simulink model "OFDMTxRx221121"  (R2017b)
settings: Solver=VariableStepAuto  StartTime=0.0  StopTime=10  RelTol=1e-3
InitFcn:
  | Ts = 1e-6;
  | simParams.Ts = Ts;
  | simParams.TsTx = Ts;
  | simParams.TsRx = Ts;
  | simParams.nFFT = 1024;
  | simParams.lengthCP = 128;
  | nFFT = simParams.nFFT;
  | simParams.NSubcarriers = 398;
  | simParams.windowing = 16;
undefined symbols (not defined in the file): fft_size, i
libraries: hdlsllib x34, simulink x26, simulink_need_slupdate x17, dspmathops x5, dspxfrm3 x3, dspsigops x2, commdigbbndam3 x1, commrflib2 x1, commseqgen3 x1
(part 1 of 2)
settings Model: PauseTimes=1  Creator=Pigrit  LastModifiedBy=trainee

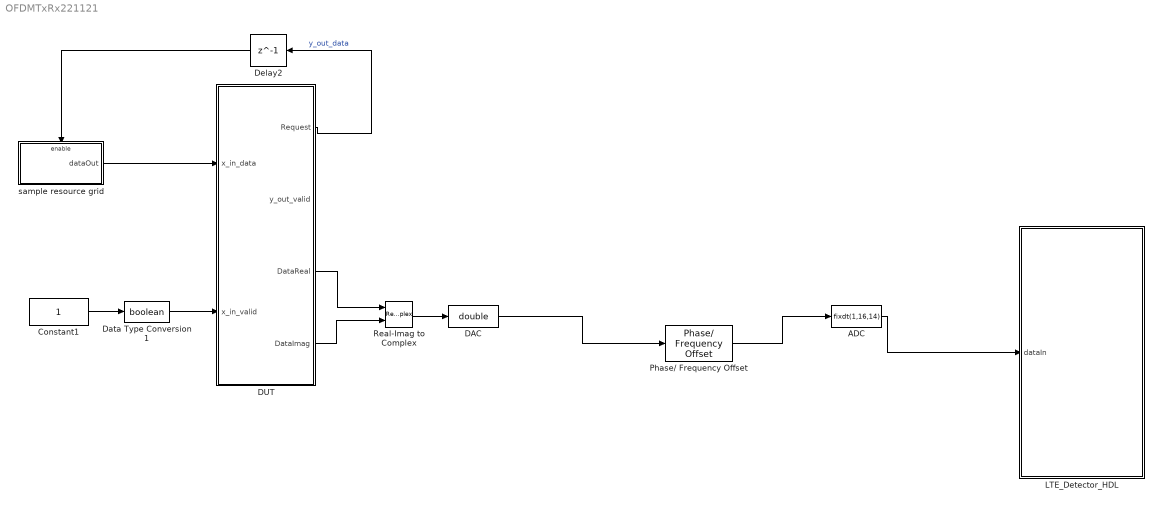
== system OFDMTxRx221121 ==
  ADC : DataTypeConversion  OutDataTypeStr=fixdt(1,16,14)  RndMeth=Nearest
  Constant1 : Constant  OutDataTypeStr=boolean  SampleTime=simParams.Ts
  DAC : DataTypeConversion  OutDataTypeStr=double  RndMeth=Nearest
  DUT : Subsystem  TreatAsAtomicUnit=on
  Data Type Conversion1 : DataTypeConversion  OutDataTypeStr=boolean
  Delay2 : Delay  DelayLength=1  InitialCondition=0  InputProcessing=Columns as channels (frame based)
  LTE_Detector_HDL : Subsystem
  Phase/ Frequency Offset : commrflib2/Phase// Frequency Offset  phaseOffset=0  freqPort=off  freqOffset=0
      settings: SourceProductName=Communications System Toolbox
  Real-Imag to Complex : RealImagToComplex
  sample resource grid : Subsystem
  wires:
  DUT/3(DataReal) -> Real-Imag to Complex/1
  Delay2/1 -> sample resource grid/Enable
  Data Type Conversion1/1 -> DUT/2(x_in_valid)
  Constant1/1 -> Data Type Conversion1/1
  DUT/1(Request) -> Delay2/1  "y_out_data"
  sample resource grid/1(dataOut) -> DUT/1(x_in_data)
  DUT/4(DataImag) -> Real-Imag to Complex/2
  Real-Imag to Complex/1 -> DAC/1
  ADC/1 -> LTE_Detector_HDL/1(dataIn)
  Phase/ Frequency Offset/1 -> ADC/1
  DAC/1 -> Phase/ Frequency Offset/1

== system OFDMTxRx221121/DUT ==
  x_in_data : Inport
  x_in_valid : Inport  Port=2
  "symmetric " : Subsystem
  Request : Outport
  y_out_valid : Outport  Port=2
  DataReal : Outport  Port=3
  DataImag : Outport  Port=4
  wires:
  x_in_valid/1 -> "symmetric "/Enable, y_out_valid/1
  x_in_data/1 -> "symmetric "/1(x_in)
  "symmetric "/1(y_out) -> Request/1
  "symmetric "/2(Data1) -> DataReal/1
  "symmetric "/3(Data2) -> DataImag/1

== system OFDMTxRx221121/LTE_Detector_HDL ==
  dataIn : Inport
  Buffer : Buffer  N=1000  OutputFrames=off
  Constellation Diagram : ConstellationDiagram
  Delay1 : Delay  DelayLength=11  InitialCondition=0
  Delay2 : Delay  DelayLength=1196  InitialCondition=0
  FFT : Subsystem
  Frequency_Correction : Subsystem
  Frequency_Correction1 : Subsystem
  Frequency_Correction2 : Subsystem
  Frequency_Estimation : Subsystem
  Frequency_Estimation1 : Subsystem
  Frequency_Estimation2 : Subsystem
  Number of subcarriers : Constant  Value=0  OutDataTypeStr=fixdt(0,12,0)  SampleTime=Ts
  Scope : Scope  NumInputPorts=3
  Spectrum Analyzer : SpectrumAnalyzer
  Переформирование отсчетов : Subsystem
  Подстройка по фазе : Subsystem
  Стробирование сигнала на nFFT отсчетов : Subsystem
  Эквалайзинг забита только формула : Subsystem
  wires:
  Стробирование сигнала на nFFT отсчетов/1(dataOut) -> FFT/1(dataIn)
  Стробирование сигнала на nFFT отсчетов/2(ValidOut) -> FFT/2(validIn)
  Buffer/1 -> Constellation Diagram/1
  Переформирование отсчетов/3(AngOut) -> Подстройка по фазе/2(AngIn)
  Переформирование отсчетов/4(ValidOut) -> Подстройка по фазе/3("ValidIn "), Эквалайзинг забита только формула/2("ValidIn ")
  Подстройка по фазе/1(Out1) -> Buffer/1
  Переформирование отсчетов/1("PureSig ") -> Подстройка по фазе/1(PureSigIn)
  dataIn/1 -> Spectrum Analyzer/1, Delay2/1, Frequency_Estimation1/1(data)
  FFT/1(dataOut) -> Переформирование отсчетов/1(In1)
  FFT/2(validOut) -> Переформирование отсчетов/2(In2)
  Переформирование отсчетов/2(MagOut) -> Эквалайзинг забита только формула/1(MagIn)
  Frequency_Estimation1/2(MiddlePoint) -> Scope/2, Delay1/1
  Delay2/1 -> Scope/3, Frequency_Correction1/1(dataIn)
  Frequency_Correction1/1(dataOut) -> Стробирование сигнала на nFFT отсчетов/1(In1)
  Delay1/1 -> Стробирование сигнала на nFFT отсчетов/2(In2)
  Frequency_Estimation1/1(freqEst) -> Scope/1, Frequency_Correction1/2(freq)

== system OFDMTxRx221121/sample resource grid ==
  request1 : EnablePort
  PN Sequence Generator : commseqgen3/PN Sequence Generator  poly='z^23+z^21+z^17 + z^11 + z^5 +1'  ini_sta=[0 1 1 0 0 1 0 0 0 0 1 0 1 1 0 0 1 0 0 1 0 0 1]  outBitMaskSource=Dialog parameter  shift=0  outVarSiz=off  maxOutSizeMode=Dialog parameter  maxOutSize=[10 1]  Ts=simParams.Ts  sampPerFrame=1  reset=off  bitPackedOutputs=on  outDataType=boolean  numPackedBits=6  bitPackDataSigned=off  bitPackedOutDType=Smallest integer
      settings: SourceProductName=Communications System Toolbox
  dataOut : Outport
  wires:
  PN Sequence Generator/1 -> dataOut/1

== system OFDMTxRx221121/DUT/symmetric  ==
  x_in : Inport
  Enable : EnablePort
  Add CP and windowing : Subsystem
  Complex to Real-Imag : ComplexToRealImag
  IFFT : Subsystem
  Scope : Scope  NumInputPorts=2
  Scope1 : Scope  NumInputPorts=2
  fORM1 : Subsystem
  y_out1 : Scope  NumInputPorts=2
  "Сдвиг в симметричный вид " : Subsystem
  y_out : Outport  InitialOutput=0
  Data1 : Outport  Port=2  InitialOutput=0
  Data2 : Outport  Port=3  InitialOutput=0
  wires:
  fORM1/1(dataRequest) -> y_out/1
  x_in/1 -> fORM1/1(dataIn)
  Add CP and windowing/1(Out1) -> Complex to Real-Imag/1
  Complex to Real-Imag/1 -> Data2/1
  IFFT/1(dataOut) -> Scope/1, Add CP and windowing/1(In1)
  Complex to Real-Imag/2 -> Data1/1
  "Сдвиг в симметричный вид "/1(dataOut) -> Scope1/1, IFFT/1(dataIn)
  "Сдвиг в симметричный вид "/2(validOut) -> Scope1/2, IFFT/2(validIn)
  IFFT/2(validOut) -> Scope/2, Add CP and windowing/2(In2)
  fORM1/2(dataOut) -> y_out1/1, "Сдвиг в симметричный вид "/1(dataIn)
  fORM1/3(validOut) -> y_out1/2, "Сдвиг в симметричный вид "/2(validIn)

== system OFDMTxRx221121/LTE_Detector_HDL/FFT ==
  note: Set input of FFT to input wordlength + FFT growth to allow
      | the output of the FFT to scale. Maximum bit growth is equal
      | to log2(nFFT).
  dataIn : Inport
  validIn : Inport  Port=2
  Data Type Conversion : DataTypeConversion  OutDataTypeStr=fixdt(1,18,10)  RndMeth=Round
  Delay{1..2,4..5} (4 alike) : Delay  DelayLength=1  InitialCondition=0  InputProcessing=Columns as channels (frame based)
  FFT HDL Optimized : dspxfrm3/FFT HDL Optimized  FFTLength=1024  Architecture=Streaming Radix 2^2  ComplexMultiplication=Use 3 multipliers and 5 adders  BitReversedOutput=off  BitReversedInput=off  Normalize=off  SimulateUsing=Code generation  RoundingMethod=Floor  ResetInputPort=off  StartOutputPort=off  EndOutputPort=off
      settings: SourceProductName=DSP System Toolbox  SourceProductBaseCode=DS
  Signal Specification : SignalSpecification  Dimensions=1
  Signal Specification1 : SignalSpecification  Dimensions=1
  dataOut : Outport
  validOut : Outport  Port=2
  wires:
  Signal Specification1/1 -> FFT HDL Optimized/2
  Signal Specification/1 -> FFT HDL Optimized/1
  FFT HDL Optimized/2 -> Delay5/1
  FFT HDL Optimized/1 -> Delay4/1
  Delay4/1 -> Data Type Conversion/1
  Delay2/1 -> Signal Specification1/1
  dataIn/1 -> Delay1/1
  validIn/1 -> Delay2/1
  Delay1/1 -> Signal Specification/1
  Data Type Conversion/1 -> dataOut/1
  Delay5/1 -> validOut/1

== system OFDMTxRx221121/LTE_Detector_HDL/Frequency_Correction ==
  note: This subsystem corrects the frequency offset using an Numerically Controller Oscillator (NCO) and a conjugate multiplication.
  dataIn : Inport
  freq : Inport  Port=2
  Data Type Conversion : DataTypeConversion  OutDataTypeStr=fixdt(1,16,15)  RndMeth=Nearest
  Delay{1..6} (6 alike) : Delay  DelayLength=1  InitialCondition=0  UseCircularBuffer=on
  Gain : Gain  Gain=2^9  OutDataTypeStr=int16
  NCO HDL Optimized : dspsigops/NCO HDL Optimized  PhaseIncrementSource=Input port  PhaseIncrement=100  PhaseOffsetSource=Property  PhaseOffset=0  DitherSource=Property  NumDitherBits=4  PhaseQuantization=on  NumQuantizerAccumulatorBits=12  LUTCompress=on  ResetAction=off  ValidInputPort=off  Waveform=Complex exponential  PhasePort=off  SimulateUsing=Code generation  AccumulatorWL=16  OutputDataType=Binary point scaling  OutputWL=16  OutputFL=14
      settings: SourceProductName=DSP System Toolbox  SourceProductBaseCode=DS
  Product1 : Product
  Scope : Scope  NumInputPorts=2
  Signal Spec : SignalSpecification  Dimensions=1
  Unit Delay Enabled : simulink_need_slupdate/Unit Delay Enabled  vinit=0.0  tsamp=-1
      settings: SourceProductName=Simulink  SourceProductBaseCode=SL
  complexConjugate : Math  Operator=conj  SaturateOnIntegerOverflow=on
  dataOut : Outport
  wires:
  complexConjugate/1 -> Delay3/1
  NCO HDL Optimized/2 -> Unit Delay Enabled/2
  dataIn/1 -> Delay2/1
  Product1/1 -> Delay4/1
  NCO HDL Optimized/1 -> Unit Delay Enabled/1
  Unit Delay Enabled/1 -> complexConjugate/1
  Data Type Conversion/1 -> Delay1/1
  Delay2/1 -> Scope/2, Product1/1
  Delay1/1 -> dataOut/1
  Delay4/1 -> Data Type Conversion/1
  Delay3/1 -> Scope/1, Product1/2
  Gain/1 -> Delay5/1
  freq/1 -> Delay6/1
  Delay6/1 -> Gain/1
  Signal Spec/1 -> NCO HDL Optimized/1
  Delay5/1 -> Signal Spec/1

== system OFDMTxRx221121/LTE_Detector_HDL/Frequency_Correction1 ==
  note: This subsystem corrects the frequency offset using an Numerically Controller Oscillator (NCO) and a conjugate multiplication.
  dataIn : Inport
  freq : Inport  Port=2
  Data Type Conversion : DataTypeConversion  OutDataTypeStr=fixdt(1,16,15)  RndMeth=Nearest
  Delay{1..6} (6 alike) : Delay  DelayLength=1  InitialCondition=0  UseCircularBuffer=on
  Gain : Gain  Gain=2^9  OutDataTypeStr=int16
  NCO HDL Optimized : dspsigops/NCO HDL Optimized  PhaseIncrementSource=Input port  PhaseIncrement=100  PhaseOffsetSource=Property  PhaseOffset=0  DitherSource=Property  NumDitherBits=4  PhaseQuantization=on  NumQuantizerAccumulatorBits=12  LUTCompress=on  ResetAction=off  ValidInputPort=off  Waveform=Complex exponential  PhasePort=off  SimulateUsing=Code generation  AccumulatorWL=16  OutputDataType=Binary point scaling  OutputWL=16  OutputFL=14
      settings: SourceProductName=DSP System Toolbox  SourceProductBaseCode=DS
  Product1 : Product
  Scope : Scope  NumInputPorts=2
  Signal Spec : SignalSpecification  Dimensions=1
  Unit Delay Enabled : simulink_need_slupdate/Unit Delay Enabled  vinit=0.0  tsamp=-1
      settings: SourceProductName=Simulink  SourceProductBaseCode=SL
  complexConjugate : Math  Operator=conj  SaturateOnIntegerOverflow=on
  dataOut : Outport
  wires:
  complexConjugate/1 -> Delay3/1
  NCO HDL Optimized/2 -> Unit Delay Enabled/2
  dataIn/1 -> Delay2/1
  Product1/1 -> Delay4/1
  NCO HDL Optimized/1 -> Unit Delay Enabled/1
  Unit Delay Enabled/1 -> complexConjugate/1
  Data Type Conversion/1 -> Delay1/1
  Delay2/1 -> Scope/2, Product1/1
  Delay1/1 -> dataOut/1
  Delay4/1 -> Data Type Conversion/1
  Delay3/1 -> Scope/1, Product1/2
  Gain/1 -> Delay5/1
  freq/1 -> Delay6/1
  Delay6/1 -> Gain/1
  Signal Spec/1 -> NCO HDL Optimized/1
  Delay5/1 -> Signal Spec/1

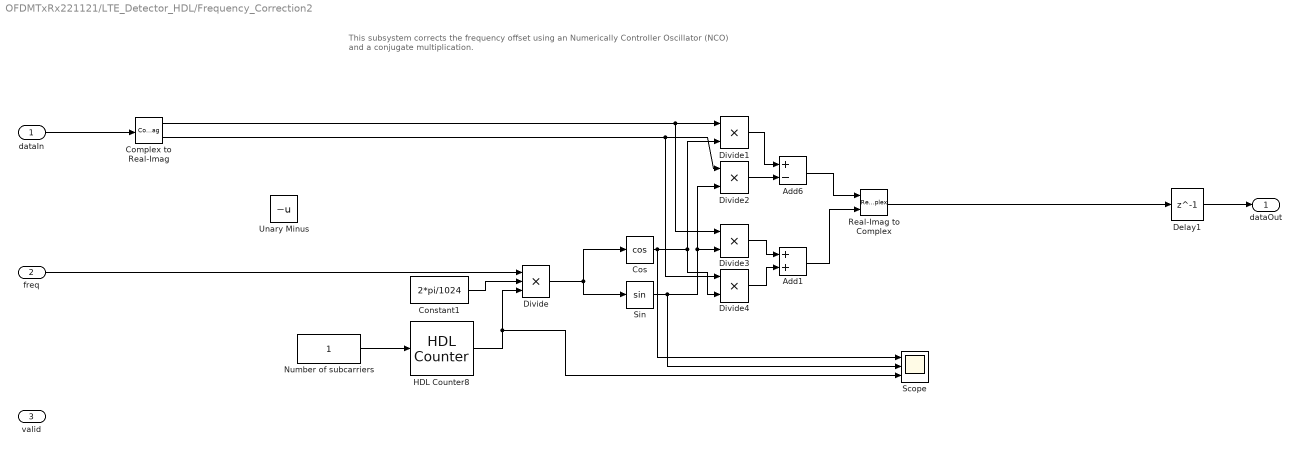
== system OFDMTxRx221121/LTE_Detector_HDL/Frequency_Correction2 ==
  note: This subsystem corrects the frequency offset using an Numerically Controller Oscillator (NCO) and a conjugate multiplication.
  dataIn : Inport
  freq : Inport  Port=2
  "valid " : Inport  Port=3
  Add1 : Sum
  Add6 : Sum  Inputs=+-
  Complex to Real-Imag : ComplexToRealImag
  Constant1 : Constant  Value=2*pi/1024  SampleTime=simParams.Ts
  Cos : Trigonometry  Operator=cos
  Delay1 : Delay  DelayLength=1  InitialCondition=0  UseCircularBuffer=on
  Divide : Product  Inputs=***  SaturateOnIntegerOverflow=on  RndMeth=Zero
  Divide{1..4} (4 alike) : Product  Inputs=**  SaturateOnIntegerOverflow=on  RndMeth=Zero
  HDL Counter8 : hdlsllib/Sources/HDL Counter  CountType=Count limited  CountInit=0  CountStep=1  CountMax=1023  CountFromType=Initial value  CountFrom=0  CountResetPort=off  CountLoadPort=off  CountEnbPort=on  CountDirPort=off  CountDataType=Unsigned  CountWordLen=11  CountFracLen=0  CountSampTime=1
      settings: SourceProductBaseCode=HD
  Number of subcarriers : Constant  OutDataTypeStr=boolean  SampleTime=Ts
  Real-Imag to Complex : RealImagToComplex
  Scope : Scope  NumInputPorts=3
  Sin : Trigonometry
  Unary Minus : UnaryMinus
  dataOut : Outport
  wires:
  Real-Imag to Complex/1 -> Delay1/1
  Delay1/1 -> dataOut/1
  dataIn/1 -> Complex to Real-Imag/1
  HDL Counter8/1 -> Scope/3, Divide/3
  Constant1/1 -> Divide/2
  Divide/1 -> Cos/1, Sin/1
  Complex to Real-Imag/1 -> Divide3/1, Divide1/1
  Cos/1 -> Scope/1, Divide4/2, Divide1/2
  Divide1/1 -> Add6/1
  Complex to Real-Imag/2 -> Divide4/1, Divide2/1
  Sin/1 -> Scope/2, Divide3/2, Divide2/2
  Divide2/1 -> Add6/2
  Divide3/1 -> Add1/1
  Divide4/1 -> Add1/2
  Add6/1 -> Real-Imag to Complex/1
  Add1/1 -> Real-Imag to Complex/2
  freq/1 -> Divide/1
  Number of subcarriers/1 -> HDL Counter8/1

== system OFDMTxRx221121/LTE_Detector_HDL/Frequency_Estimation ==
  data : Inport
  Angle_Filter : Subsystem
  Angle_at_Maximum : Subsystem
  Cyclic_Prefix_Correlator : Subsystem
  Delay14 : Delay  DelayLength=30  InitialCondition=0  UseCircularBuffer=on
  Rect_to_Polar : Subsystem
  Scope1 : Scope  NumInputPorts=2
  freqEst : Outport
  MiddlePoint : Outport  Port=2
  wires:
  Angle_at_Maximum/1(angleOut) -> Angle_Filter/1(angleIn)
  Cyclic_Prefix_Correlator/1(corrOut) -> Scope1/2, Rect_to_Polar/1(dataIn)
  Angle_at_Maximum/2(validOut) -> Delay14/1, MiddlePoint/1, Angle_Filter/2(en)
  Angle_Filter/1(angleOut) -> freqEst/1
  data/1 -> Cyclic_Prefix_Correlator/1(dataIn)
  Delay14/1 -> Scope1/1
  Rect_to_Polar/1(magOut) -> Angle_at_Maximum/1(MagIn)
  Rect_to_Polar/2(angleOut) -> Angle_at_Maximum/2(AngleIn)
  Rect_to_Polar/3(validOut) -> Angle_at_Maximum/3(ValidIn)

== system OFDMTxRx221121/LTE_Detector_HDL/Frequency_Estimation1 ==
  data : Inport
  Angle_Filter : Subsystem
  Angle_at_Maximum : Subsystem
  Angle_at_Maximum1 : Subsystem
  Cyclic_Prefix_Correlator : Subsystem
  Rect_to_Polar : Subsystem
  freqEst : Outport
  MiddlePoint : Outport  Port=2
  wires:
  Rect_to_Polar/3(validOut) -> Angle_at_Maximum/3(validIn)
  Rect_to_Polar/1(magOut) -> Angle_at_Maximum/1(magIn)
  Cyclic_Prefix_Correlator/1(corrOut) -> Rect_to_Polar/1(dataIn)
  Angle_at_Maximum/2(validOut) -> MiddlePoint/1
  Rect_to_Polar/2(angleOut) -> Angle_at_Maximum/2(angleIn)
  Angle_at_Maximum/1(angleOut) -> freqEst/1
  data/1 -> Cyclic_Prefix_Correlator/1(dataIn)

== system OFDMTxRx221121/LTE_Detector_HDL/Frequency_Estimation2 ==
  data : Inport
  Angle_at_Maximum : Subsystem
  Cyclic_Prefix_Correlator : Subsystem
  Rect_to_Polar : Subsystem
  Scope14 : Scope  NumInputPorts=3
  freqEst : Outport
  CPCorrMag : Outport  Port=2
  wires:
  data/1 -> Cyclic_Prefix_Correlator/1(dataIn)
  Rect_to_Polar/3(validOut) -> Angle_at_Maximum/3(validIn)
  Rect_to_Polar/2(angleOut) -> Scope14/2, Angle_at_Maximum/2(angleIn)
  Rect_to_Polar/1(magOut) -> CPCorrMag/1, Angle_at_Maximum/1(magIn)
  Cyclic_Prefix_Correlator/1(corrOut) -> Rect_to_Polar/1(dataIn)
  Angle_at_Maximum/1(angleOut) -> Scope14/1, freqEst/1
  Angle_at_Maximum/2(validOut) -> Scope14/3

== system OFDMTxRx221121/LTE_Detector_HDL/Переформирование отсчетов ==
  In1 : Inport
  In2 : Inport  Port=2
  Compare To Constant2 : simulink/Logic and Bit Operations/Compare To Constant  relop=<  const=512  OutDataTypeStr=boolean
  Delay1 : Delay  DelayLength=512  InitialCondition=0  InputProcessing=Columns as channels (frame based)
  Delay2 : Delay  DelayLength=22  InitialCondition=0  InputProcessing=Columns as channels (frame based)
  Delay4 : Delay  DelayLength=1024  InitialCondition=0  InputProcessing=Columns as channels (frame based)
  HDL Counter1 : hdlsllib/Sources/HDL Counter  CountType=Count limited  CountInit=0  CountStep=1  CountMax=1023  CountFromType=Initial value  CountFrom=0  CountResetPort=on  CountLoadPort=off  CountEnbPort=on  CountDirPort=off  CountDataType=Unsigned  CountWordLen=11  CountFracLen=0  CountSampTime=1
      settings: SourceProductBaseCode=HD
  Logical Operator1 : Logic  Operator=NOT  IconShape=distinctive  AllPortsSameDT=off  OutDataTypeStr=boolean
  Rect_to_Polar : Subsystem
  Signal Specification1 : SignalSpecification  Dimensions=1
  Switch4 : Switch  Criteria=u2 ~= 0
  "PureSig " : Outport
  MagOut : Outport  Port=2
  AngOut : Outport  Port=3
  ValidOut : Outport  Port=4
  wires:
  Delay4/1 -> Switch4/3
  Compare To Constant2/1 -> Switch4/2
  HDL Counter1/1 -> Compare To Constant2/1
  Logical Operator1/1 -> HDL Counter1/1
  Switch4/1 -> Delay2/1, Signal Specification1/1
  Delay1/1 -> Logical Operator1/1, HDL Counter1/2, Rect_to_Polar/2("ValidIn ")
  In2/1 -> Delay1/1
  In1/1 -> Switch4/1, Delay4/1
  Rect_to_Polar/3(validOut) -> ValidOut/1
  Rect_to_Polar/1(magOut) -> MagOut/1
  Delay2/1 -> "PureSig "/1
  Rect_to_Polar/2(angleOut) -> AngOut/1
  Signal Specification1/1 -> Rect_to_Polar/1(dataIn)

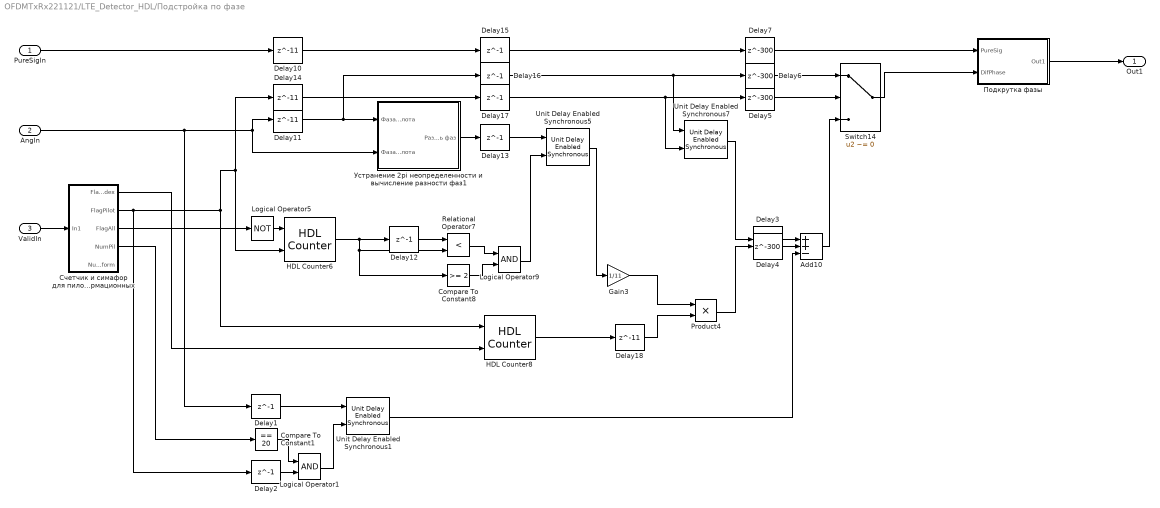
== system OFDMTxRx221121/LTE_Detector_HDL/Подстройка по фазе ==
  PureSigIn : Inport
  AngIn : Inport  Port=2
  "ValidIn " : Inport  Port=3
  Add10 : Sum  Inputs=++-
  Compare To Constant1 : simulink/Logic and Bit Operations/Compare To Constant  relop===  const=20  OutDataTypeStr=boolean
  Compare To Constant8 : simulink/Logic and Bit Operations/Compare To Constant  relop=>=  const=2  OutDataTypeStr=boolean
  Delay{1..2,12..13,15..17} (7 alike) : Delay  DelayLength=1  InitialCondition=0  UseCircularBuffer=on
  Delay{10..11,14,18} (4 alike) : Delay  DelayLength=11  InitialCondition=0  UseCircularBuffer=on
  Delay{3..7} (5 alike) : Delay  DelayLength=300  InitialCondition=0  UseCircularBuffer=on
  Gain3 : Gain  Gain=1/11
  HDL Counter6 : hdlsllib/Sources/HDL Counter  CountType=Count limited  CountInit=0  CountStep=1  CountMax=20  CountFromType=Initial value  CountFrom=0  CountResetPort=on  CountLoadPort=off  CountEnbPort=on  CountDirPort=off  CountDataType=Unsigned  CountWordLen=8  CountFracLen=0  CountSampTime=1
      settings: SourceProductBaseCode=HD
  HDL Counter8 : hdlsllib/Sources/HDL Counter  CountType=Count limited  CountInit=1  CountStep=1  CountMax=20  CountFromType=Initial value  CountFrom=1  CountResetPort=on  CountLoadPort=off  CountEnbPort=on  CountDirPort=off  CountDataType=Unsigned  CountWordLen=8  CountFracLen=0  CountSampTime=1
      settings: SourceProductBaseCode=HD
  Logical Operator1 : Logic  AllPortsSameDT=off  OutDataTypeStr=boolean
  Logical Operator5 : Logic  Operator=NOT  AllPortsSameDT=off  OutDataTypeStr=boolean
  Logical Operator9 : Logic  AllPortsSameDT=off  OutDataTypeStr=boolean
  Product4 : Product
  Relational Operator7 : RelationalOperator  Operator=<  OutDataTypeStr=boolean  RndMeth=Nearest
  Switch14 : Switch  Criteria=u2 ~= 0
  Unit Delay Enabled Synchronous1 : hdlsllib/Discrete/Unit Delay Enabled Synchronous  InitialCondition=0.0  SampleTime=-1
      settings: SourceProductName=HDL Coder  SourceProductBaseCode=HD
  Unit Delay Enabled Synchronous5 : hdlsllib/Discrete/Unit Delay Enabled Synchronous  InitialCondition=0.0  SampleTime=-1
      settings: SourceProductName=HDL Coder  SourceProductBaseCode=HD
  Unit Delay Enabled Synchronous7 : hdlsllib/Discrete/Unit Delay Enabled Synchronous  InitialCondition=0.0  SampleTime=-1
      settings: SourceProductName=HDL Coder  SourceProductBaseCode=HD
  Подкрутка фазы : Subsystem
  Счетчик и симафор для пилотов и информационных : Subsystem
  Устранение 2pi неопределенности и вычисление разности фаз1 : Subsystem
  Out1 : Outport
  wires:
  "ValidIn "/1 -> Счетчик и симафор для пилотов и информационных/1(In1)
  Delay10/1 -> Delay15/1
  Подкрутка фазы/1(Out1) -> Out1/1
  PureSigIn/1 -> Delay10/1
  Delay11/1 -> Устранение 2pi неопределенности и вычисление разности фаз1/1("Фаза \"левого\" пилота"), Delay16/1
  Switch14/1 -> Подкрутка фазы/2("DifPhase ")
  Logical Operator9/1 -> Unit Delay Enabled Synchronous5/2
  Устранение 2pi неопределенности и вычисление разности фаз1/1("Разность фаз ") -> Delay13/1
  Relational Operator7/1 -> Logical Operator9/1
  Delay16/1 -> Unit Delay Enabled Synchronous7/1, Delay6/1
  Счетчик и симафор для пилотов и информационных/3(FlagAll) -> Logical Operator5/1
  Delay15/1 -> Delay7/1
  Delay12/1 -> Relational Operator7/1
  AngIn/1 -> Delay1/1, Устранение 2pi неопределенности и вычисление разности фаз1/2("Фаза \"правого\" пилота"), Delay11/1
  Logical Operator5/1 -> HDL Counter6/1
  HDL Counter8/1 -> Delay18/1
  Delay13/1 -> Unit Delay Enabled Synchronous5/1
  Compare To Constant8/1 -> Logical Operator9/2
  Unit Delay Enabled Synchronous5/1 -> Gain3/1
  Счетчик и симафор для пилотов и информационных/1(FlagIndex) -> HDL Counter8/2
  Product4/1 -> Delay4/1
  Gain3/1 -> Product4/1
  Delay17/1 -> Unit Delay Enabled Synchronous7/2, Delay5/1
  Delay18/1 -> Product4/2
  Delay14/1 -> Delay17/1
  Add10/1 -> Switch14/3
  Unit Delay Enabled Synchronous7/1 -> Delay3/1
  HDL Counter6/1 -> Delay12/1, Relational Operator7/2, Compare To Constant8/1
  Счетчик и симафор для пилотов и информационных/4(NumPil) -> Compare To Constant1/1
  Счетчик и симафор для пилотов и информационных/2(FlagPilot) -> Delay2/1, Delay14/1, HDL Counter6/2, HDL Counter8/1
  Delay2/1 -> Logical Operator1/2
  Compare To Constant1/1 -> Logical Operator1/1
  Logical Operator1/1 -> Unit Delay Enabled Synchronous1/2
  Delay1/1 -> Unit Delay Enabled Synchronous1/1
  Unit Delay Enabled Synchronous1/1 -> Add10/3
  Delay3/1 -> Add10/1
  Delay4/1 -> Add10/2
  Delay5/1 -> Switch14/2
  Delay6/1 -> Switch14/1
  Delay7/1 -> Подкрутка фазы/1(PureSig)

== system OFDMTxRx221121/LTE_Detector_HDL/Стробирование сигнала на nFFT отсчетов ==
  In1 : Inport
  In2 : Inport  Port=2
  Compare To Constant : simulink/Logic and Bit Operations/Compare To Constant  relop=>  const=0  OutDataTypeStr=boolean
  Delay1 : Delay  DelayLength=1  InitialCondition=0
  HDL Counter : hdlsllib/Sources/HDL Counter  CountType=Count limited  CountInit=0  CountStep=1  CountMax=1023  CountFromType=Initial value  CountFrom=0  CountResetPort=off  CountLoadPort=off  CountEnbPort=on  CountDirPort=off  CountDataType=Unsigned  CountWordLen=11  CountFracLen=0  CountSampTime=1
      settings: SourceProductBaseCode=HD
  Logical Operator1 : Logic  IconShape=distinctive  AllPortsSameDT=off  OutDataTypeStr=boolean
  Logical Operator4 : Logic  Operator=OR  IconShape=distinctive  AllPortsSameDT=off  OutDataTypeStr=boolean
  dataOut : Outport
  ValidOut : Outport  Port=2
  wires:
  Logical Operator4/1 -> Delay1/1, HDL Counter/1, ValidOut/1
  HDL Counter/1 -> Compare To Constant/1
  Logical Operator1/1 -> Logical Operator4/2
  Delay1/1 -> Logical Operator1/2
  Compare To Constant/1 -> Logical Operator1/1
  In1/1 -> dataOut/1
  In2/1 -> Logical Operator4/1

== system OFDMTxRx221121/LTE_Detector_HDL/Эквалайзинг забита только формула ==
  MagIn : Inport
  "ValidIn " : Inport  Port=2
  2interp : Subsystem
  Constant1 : Constant  Value=3
  Delay1 : Delay  DelayLength=11  InitialCondition=0  UseCircularBuffer=on
  Delay6 : Delay  DelayLength=21  InitialCondition=0  UseCircularBuffer=on
  Divide : Product  Inputs=*/  SaturateOnIntegerOverflow=on  RndMeth=Zero
  Счетчик и симафор для пилотов и информационных : Subsystem
  Out1 : Outport
  wires:
  "ValidIn "/1 -> Счетчик и симафор для пилотов и информационных/1(In1)
  Constant1/1 -> Divide/1
  MagIn/1 -> Divide/2
  Divide/1 -> 2interp/3(y3), Delay6/1, Delay1/1
  Delay6/1 -> 2interp/1(y1)
  Delay1/1 -> 2interp/2(y2)

== system OFDMTxRx221121/DUT/symmetric /Add CP and windowing ==
  In1 : Inport
  In2 : Inport  Port=2
  Compare To Constant : simulink/Logic and Bit Operations/Compare To Constant  relop=>=  const=896  OutDataTypeStr=boolean
  Delay1 : Delay  DelayLength=1024
  Delay2 : Delay  DelayLength=1024
  FFT : Subsystem
  HDL Counter : hdlsllib/Sources/HDL Counter  CountType=Count limited  CountInit=0  CountStep=1  CountMax=1023  CountFromType=Initial value  CountFrom=0  CountResetPort=on  CountLoadPort=off  CountEnbPort=on  CountDirPort=off  CountDataType=Unsigned  CountWordLen=10  CountFracLen=0  CountSampTime=1
      settings: SourceProductBaseCode=HD
  Logical Operator2 : Logic  Operator=NOT  AllPortsSameDT=off  OutDataTypeStr=boolean
  Scope : Scope
  Switch1 : Switch  Criteria=u2 > Threshold
  y_out2 : Scope  NumInputPorts=3
  Out1 : Outport
  wires:
  Delay1/1 -> y_out2/2, Switch1/3
  HDL Counter/1 -> Compare To Constant/1
  Compare To Constant/1 -> Switch1/2
  Logical Operator2/1 -> HDL Counter/1
  Switch1/1 -> FFT/1(dataIn), y_out2/1, Out1/1
  In1/1 -> Delay1/1, Switch1/1
  In2/1 -> Delay2/1, Logical Operator2/1, HDL Counter/2
  Delay2/1 -> FFT/2(validIn), y_out2/3
  FFT/1(dataOut) -> Scope/1

== system OFDMTxRx221121/DUT/symmetric /IFFT ==
  note: Set input of FFT to input wordlength + FFT growth to allow
      | the output of the FFT to scale. Maximum bit growth is equal
      | to log2(nFFT).
  dataIn : Inport
  validIn : Inport  Port=2
  Data Type Conversion : DataTypeConversion  OutDataTypeStr=fixdt(1,23,15)  RndMeth=Nearest
  Delay{1..2,4..5} (4 alike) : Delay  DelayLength=1  InitialCondition=0  InputProcessing=Columns as channels (frame based)
  IFFT HDL Optimized : dspxfrm3/IFFT HDL Optimized  FFTLength=simParams.nFFT  Architecture=Streaming Radix 2^2  ComplexMultiplication=Use 3 multipliers and 5 adders  BitReversedOutput=off  BitReversedInput=off  Normalize=on  SimulateUsing=Code generation  RoundingMethod=Floor  ResetInputPort=off  StartOutputPort=off  EndOutputPort=off
      settings: SourceProductName=DSP System Toolbox  SourceProductBaseCode=DS
  Signal Specification : SignalSpecification  Dimensions=1
  Signal Specification1 : SignalSpecification  Dimensions=1
  dataOut : Outport
  validOut : Outport  Port=2
  wires:
  validIn/1 -> Delay2/1
  dataIn/1 -> Delay1/1
  Delay4/1 -> dataOut/1
  Delay2/1 -> Signal Specification1/1
  IFFT HDL Optimized/1 -> Delay4/1
  IFFT HDL Optimized/2 -> Delay5/1
  Signal Specification/1 -> IFFT HDL Optimized/1
  Signal Specification1/1 -> IFFT HDL Optimized/2
  Data Type Conversion/1 -> Signal Specification/1
  Delay1/1 -> Data Type Conversion/1
  Delay5/1 -> validOut/1

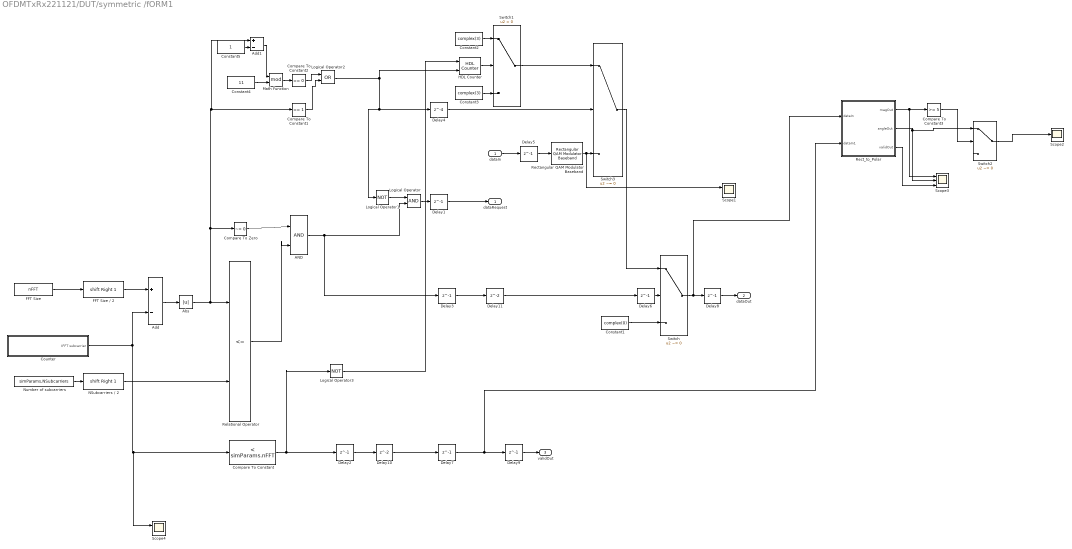
== system OFDMTxRx221121/DUT/symmetric /fORM1 ==
  dataIn : Inport
  AND : Logic  IconShape=distinctive  AllPortsSameDT=off  OutDataTypeStr=boolean
  Abs : Abs
  Add : Sum  Inputs=+-  OutDataTypeStr=fixdt(1,16,0)
  Add1 : Sum  Inputs=+-
  Compare To Constant : simulink/Logic and Bit Operations/Compare To Constant  relop=<  const=simParams.nFFT  OutDataTypeStr=boolean
  Compare To Constant1 : simulink/Logic and Bit Operations/Compare To Constant  relop===  const=1  OutDataTypeStr=boolean
  Compare To Constant2 : simulink/Logic and Bit Operations/Compare To Constant  relop===  const=0  OutDataTypeStr=boolean
  Compare To Constant3 : simulink/Logic and Bit Operations/Compare To Constant  relop=>=  const=5  OutDataTypeStr=boolean
  Compare To Zero : simulink/Logic and Bit Operations/Compare To Zero  relop=~=  OutDataTypeStr=boolean
  Constant1 : Constant  Value=complex(0)  OutDataTypeStr=fixdt(1,16,14)  SampleTime=simParams.Ts
  Constant2 : Constant  Value=complex(3)  OutDataTypeStr=fixdt(1,16,11)  SampleTime=simParams.Ts
  Constant3 : Constant  Value=complex(3)  OutDataTypeStr=fixdt(1,16,11)  SampleTime=simParams.Ts
  Constant4 : Constant  Value=11  OutDataTypeStr=int16  SampleTime=simParams.Ts
  Constant5 : Constant  OutDataTypeStr=int16  SampleTime=simParams.Ts
  "Counter " : Subsystem
  Delay{1..3,5..9} (8 alike) : Delay  DelayLength=1  InitialCondition=0  InputProcessing=Columns as channels (frame based)
  Delay10 : Delay  InitialCondition=0  InputProcessing=Columns as channels (frame based)
  Delay11 : Delay  InitialCondition=0  InputProcessing=Columns as channels (frame based)
  Delay4 : Delay  DelayLength=4  InitialCondition=0  InputProcessing=Columns as channels (frame based)
  FFT Size : Constant  Value=nFFT  OutDataTypeStr=fixdt(0,ceil(log2(simParams.nFFT))+1,0)  SampleTime=Ts
  FFT Size / 2 : ArithShift  BitShiftNumber=1  BitShiftDirection=Right
  HDL Counter : hdlsllib/Sources/HDL Counter  CountType=Count limited  CountInit=0  CountStep=1  CountMax=1  CountFromType=Initial value  CountFrom=0  CountResetPort=on  CountLoadPort=off  CountEnbPort=on  CountDirPort=off  CountDataType=Unsigned  CountWordLen=1  CountFracLen=0  CountSampTime=1
      settings: SourceProductBaseCode=HD
  Logical Operator : Logic  AllPortsSameDT=off  OutDataTypeStr=boolean
  Logical Operator1 : Logic  Operator=NOT  Inputs=1  AllPortsSameDT=off  OutDataTypeStr=boolean
  Logical Operator2 : Logic  Operator=OR  AllPortsSameDT=off  OutDataTypeStr=boolean
  Logical Operator3 : Logic  Operator=NOT  Inputs=1  AllPortsSameDT=off  OutDataTypeStr=boolean
  Math Function : Math  Operator=mod  RndMeth=Zero  SaturateOnIntegerOverflow=on
  NSubcarriers / 2 : ArithShift  BitShiftNumber=1  BitShiftDirection=Right
  Number of subcarriers : Constant  Value=simParams.NSubcarriers  OutDataTypeStr=fixdt(0,12,0)  SampleTime=Ts
  Rect_to_Polar : Subsystem
  Rectangular QAM Modulator Baseband : commdigbbndam3/Rectangular QAM Modulator Baseband  M=64  InType=Integer  Enc=Gray  Mapping=[0:15]  PowType=Min. distance between symbols  MinDist=2  AvgPow=1  PeakPow=1  Ph=0  outDtype=Fixed-point  outWordLen=16  outUDDataType=sfix(16)  outFracLenMode=User-defined  outFracLen=10  outDataTypeStr=fixdt(1,16,10)  outLastDataTypeStr=fixdt(1,16,10)
  Relational Operator : RelationalOperator  Operator=<=  OutDataTypeStr=boolean  RndMeth=Nearest
  Scope1 : Scope  NumInputPorts=2
  Scope2 : Scope
  Scope3 : Scope  NumInputPorts=3
  Scope4 : Scope  NumInputPorts=2
  Switch : Switch  Criteria=u2 ~= 0
  Switch1 : Switch  Criteria=u2 > Threshold
  Switch2 : Switch  Criteria=u2 ~= 0
  Switch3 : Switch  Criteria=u2 ~= 0
  dataRequest : Outport
  dataOut : Outport  Port=2
  validOut : Outport  Port=3
  wires:
  Switch/1 -> Rect_to_Polar/1(dataIn), Delay8/1
  Switch1/1 -> Switch3/1
  Delay4/1 -> Switch3/2
  Logical Operator/1 -> Delay1/1
  NSubcarriers / 2/1 -> Relational Operator/2
  Delay7/1 -> Rect_to_Polar/2(dataIn1), Delay9/1
  Delay6/1 -> Switch/2
  Constant2/1 -> Switch1/1
  Relational Operator/1 -> AND/2
  Compare To Zero/1 -> AND/1
  Delay1/1 -> dataRequest/1
  FFT Size/1 -> FFT Size / 2/1
  AND/1 -> Logical Operator/2, Delay3/1
  Add/1 -> Abs/1
  Constant1/1 -> Switch/3
  Delay3/1 -> Delay11/1
  Delay2/1 -> Delay10/1
  Logical Operator1/1 -> Logical Operator/1
  Constant3/1 -> Switch1/3
  dataIn/1 -> Delay5/1
  Switch3/1 -> Switch/1
  "Counter "/1(IFFT subcarrier) -> Add/2, Scope4/1, Compare To Constant/1
  Delay9/1 -> validOut/1
  Delay10/1 -> Delay7/1
  Delay8/1 -> dataOut/1
  Number of subcarriers/1 -> NSubcarriers / 2/1
  FFT Size / 2/1 -> Add/1
  HDL Counter/1 -> Switch1/2
  Delay11/1 -> Delay6/1
  Compare To Constant2/1 -> Logical Operator2/1
  Rectangular QAM Modulator Baseband/1 -> Scope1/1, Switch3/3
  Delay5/1 -> Rectangular QAM Modulator Baseband/1
  Abs/1 -> Add1/1, Compare To Constant1/1, Compare To Zero/1, Relational Operator/1
  Constant4/1 -> Math Function/2
  Math Function/1 -> Compare To Constant2/1
  Compare To Constant/1 -> Logical Operator3/1, Delay2/1
  Logical Operator3/1 -> HDL Counter/1
  Rect_to_Polar/3(validOut) -> Scope3/3
  Switch2/1 -> Scope2/1
  Rect_to_Polar/1(magOut) -> Scope3/1, Compare To Constant3/1
  Rect_to_Polar/2(angleOut) -> Switch2/1, Scope3/2
  Compare To Constant3/1 -> Switch2/2
  Compare To Constant1/1 -> Logical Operator2/2
  Logical Operator2/1 -> Logical Operator1/1, Delay4/1, HDL Counter/2
  Add1/1 -> Math Function/1
  Constant5/1 -> Add1/2

== system OFDMTxRx221121/DUT/symmetric /Сдвиг в симметричный вид  ==
  note: Count 2 full FFT frames
  note: If a full IFFT frame OR 2 full FFT frames have been counted and written into RAM, enable reading from RAM.
  note: Compensate for RAM latency
  dataIn : Inport
  validIn : Inport  Port=2
  " " : simulink/Logic and Bit Operations/Compare To Constant  relop===  const=2*simParams.nFFT-1  OutDataTypeStr=boolean
  " " : simulink/Logic and Bit Operations/Compare To Constant  relop===  const=simParams.nFFT-1  OutDataTypeStr=boolean
  Compute_Read_Address : Subsystem
  Data Type Conversion : DataTypeConversion  OutDataTypeStr=fixdt(0,log2(simParams.nFFT)+1,0)
  Data Type Conversion1 : DataTypeConversion  OutDataTypeStr=fixdt(0,log2(simParams.nFFT)+1,0)
  Delay{,1..4} (5 alike) : Delay  DelayLength=1
  Dual Port RAM : hdlsllib/HDL RAMs/Dual Port RAM  ram_size=log2(simParams.nFFT)+1
      settings: SourceProductName=HDL Coder  SourceProductBaseCode=HD
  HDL Counter : hdlsllib/Sources/HDL Counter  CountType=Count limited  CountInit=0  CountStep=1  CountMax=simParams.nFFT*2-1  CountFromType=Initial value  CountFrom=0  CountResetPort=off  CountLoadPort=off  CountEnbPort=on  CountDirPort=off  CountDataType=Unsigned  CountWordLen=log2(simParams.nFFT)+1  CountFracLen=0  CountSampTime=1
      settings: SourceProductBaseCode=HD
  Logical Operator : Logic  Operator=OR  IconShape=distinctive  AllPortsSameDT=off  OutDataTypeStr=boolean
  Scope : Scope  NumInputPorts=2
  Scope1 : Scope
  Terminator : Terminator
  dataOut : Outport
  validOut : Outport  Port=2
  wires:
  validIn/1 -> Delay3/1
  dataIn/1 -> Delay4/1
  Data Type Conversion1/1 -> Dual Port RAM/4
  Data Type Conversion/1 -> Dual Port RAM/2
  Dual Port RAM/1 -> Terminator/1
  " "/1 -> Logical Operator/1
  " "/1 -> Logical Operator/2
  Dual Port RAM/2 -> Delay2/1
  Logical Operator/1 -> Compute_Read_Address/1(rdEnable)
  Compute_Read_Address/2(rdValid) -> Delay/1
  Delay/1 -> Delay1/1
  Delay1/1 -> validOut/1
  Delay2/1 -> dataOut/1
  Delay3/1 -> Dual Port RAM/3, HDL Counter/1
  Delay4/1 -> Dual Port RAM/1
  Compute_Read_Address/1(rdAddr) -> Scope/2, Data Type Conversion1/1
  HDL Counter/1 -> Scope1/1, " "/1, " "/1, Data Type Conversion/1

== system OFDMTxRx221121/LTE_Detector_HDL/Frequency_Estimation/Angle_Filter ==
  note: This subsystem implements a 1-pole IIR filter to perform further averaging of the correlation angle results. The filter's gain is normalized to 0dB and an efficient implementation which requires only 1 multiplier is used.
  angleIn : Inport
  en : Inport  Port=2
  Add : Sum  Inputs=|-+
  Add1 : Sum  Inputs=|-+
  Data Type Conversion : DataTypeConversion
  Data Type Conversion1 : DataTypeConversion
  Delay1 : Delay  DelayLength=1  InitialCondition=0  UseCircularBuffer=on
  Delay2 : Delay  DelayLength=1  InitialCondition=0  UseCircularBuffer=on
  Delay3 : Delay  DelayLength=1  InitialCondition=0  UseCircularBuffer=on
  Gain : Gain  Gain=2^-2  OutDataTypeStr=Inherit: Same as input
  Unit Delay Enabled : simulink_need_slupdate/Unit Delay Enabled  vinit=0.0  tsamp=-1
      settings: SourceProductName=Simulink  SourceProductBaseCode=SL
  angleOut : Outport
  wires:
  angleIn/1 -> Delay2/1
  Add/1 -> Data Type Conversion/1
  Gain/1 -> Add1/1
  Unit Delay Enabled/1 -> Add1/2, Delay1/1, Add/2
  Add1/1 -> Data Type Conversion1/1
  en/1 -> Delay3/1
  Delay1/1 -> angleOut/1
  Delay2/1 -> Add/1
  Delay3/1 -> Unit Delay Enabled/2
  Data Type Conversion/1 -> Gain/1
  Data Type Conversion1/1 -> Unit Delay Enabled/1

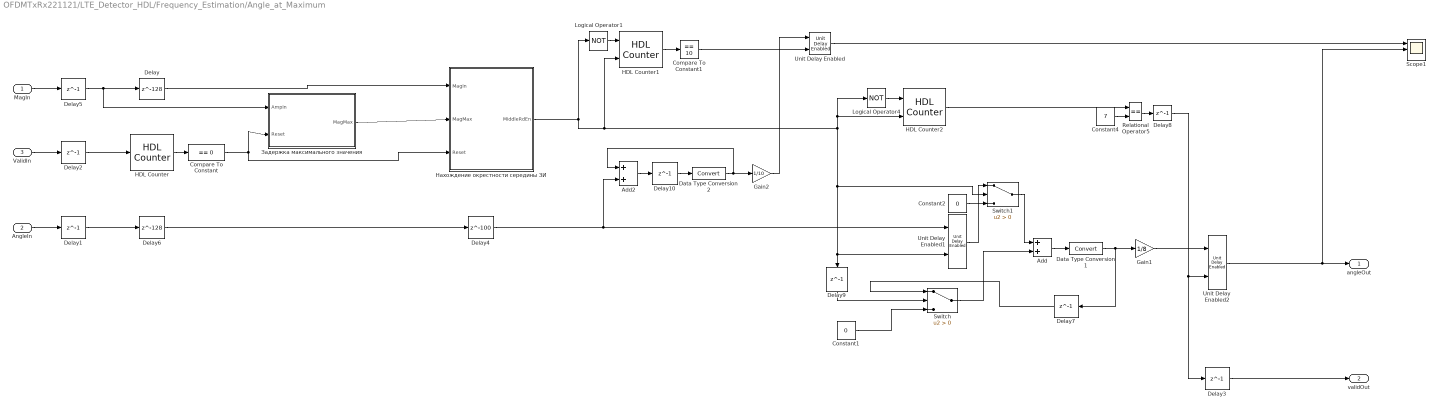
== system OFDMTxRx221121/LTE_Detector_HDL/Frequency_Estimation/Angle_at_Maximum ==
  MagIn : Inport
  AngleIn : Inport  Port=2
  ValidIn : Inport  Port=3
  Add : Sum
  Add2 : Sum  AccumDataTypeStr=fixdt(1,27,27)
  Compare To Constant : simulink/Logic and Bit Operations/Compare To Constant  relop===  const=0  OutDataTypeStr=boolean
  Compare To Constant1 : simulink/Logic and Bit Operations/Compare To Constant  relop===  const=10  OutDataTypeStr=boolean
  Constant1 : Constant  Value=0
  Constant2 : Constant  Value=0
  Constant4 : Constant  Value=7
  Data Type Conversion1 : DataTypeConversion
  Data Type Conversion2 : DataTypeConversion
  Delay : Delay  DelayLength=128  InitialCondition=0  UseCircularBuffer=on
  Delay{1..3,5,7..10} (8 alike) : Delay  DelayLength=1  InitialCondition=0  UseCircularBuffer=on
  Delay4 : Delay  DelayLength=100  InitialCondition=0  UseCircularBuffer=on
  Delay6 : Delay  DelayLength=128  InitialCondition=0  UseCircularBuffer=on
  Gain1 : Gain  Gain=1/8
  Gain2 : Gain  Gain=1/10  OutDataTypeStr=fixdt(1,24,23)
  HDL Counter : hdlsllib/Sources/HDL Counter  CountType=Count limited  CountInit=0  CountStep=1  CountMax=1152  CountFromType=Initial value  CountFrom=0  CountResetPort=off  CountLoadPort=off  CountEnbPort=on  CountDirPort=off  CountDataType=Unsigned  CountWordLen=11  CountFracLen=0  CountSampTime=1
      settings: SourceProductBaseCode=HD
  HDL Counter1 : hdlsllib/Sources/HDL Counter  CountType=Count limited  CountInit=0  CountStep=1  CountMax=40  CountFromType=Initial value  CountFrom=0  CountResetPort=on  CountLoadPort=off  CountEnbPort=on  CountDirPort=off  CountDataType=Unsigned  CountWordLen=6  CountFracLen=0  CountSampTime=1
      settings: SourceProductBaseCode=HD
  HDL Counter2 : hdlsllib/Sources/HDL Counter  CountType=Count limited  CountInit=0  CountStep=1  CountMax=7  CountFromType=Initial value  CountFrom=0  CountResetPort=on  CountLoadPort=off  CountEnbPort=on  CountDirPort=off  CountDataType=Unsigned  CountWordLen=3  CountFracLen=0  CountSampTime=1
      settings: SourceProductBaseCode=HD
  Logical Operator1 : Logic  Operator=NOT  IconShape=distinctive  AllPortsSameDT=off  OutDataTypeStr=boolean
  Logical Operator4 : Logic  Operator=NOT  IconShape=distinctive  AllPortsSameDT=off  OutDataTypeStr=boolean
  Relational Operator5 : RelationalOperator  Operator===  OutDataTypeStr=boolean  RndMeth=Nearest
  Scope1 : Scope  NumInputPorts=3
  Switch : Switch  Criteria=u2 > Threshold
  Switch1 : Switch  Criteria=u2 > Threshold
  Unit Delay Enabled : simulink_need_slupdate/Unit Delay Enabled  vinit=0.0  tsamp=-1
      settings: SourceProductName=Simulink  SourceProductBaseCode=SL
  Unit Delay Enabled1 : simulink_need_slupdate/Unit Delay Enabled  vinit=0.0  tsamp=-1
      settings: SourceProductName=Simulink  SourceProductBaseCode=SL
  Unit Delay Enabled2 : simulink_need_slupdate/Unit Delay Enabled  vinit=0.0  tsamp=-1
      settings: SourceProductName=Simulink  SourceProductBaseCode=SL
  Задержка максимального значения : Subsystem
  Нахождение окрестности середины ЗИ : Subsystem
  angleOut : Outport
  validOut : Outport  Port=2
  wires:
  Switch/1 -> Add/2
  Delay3/1 -> validOut/1
  Constant1/1 -> Switch/3
  Delay7/1 -> Switch/1
  Unit Delay Enabled1/1 -> Switch1/1
  Relational Operator5/1 -> Delay8/1
  Delay8/1 -> Unit Delay Enabled2/2, Delay3/1
  Switch1/1 -> Add/1
  Constant2/1 -> Switch1/3
  HDL Counter/1 -> Compare To Constant/1
  Add/1 -> Data Type Conversion1/1
  Delay6/1 -> Delay4/1
  Logical Operator4/1 -> HDL Counter2/1
  Unit Delay Enabled2/1 -> Scope1/2, angleOut/1
  Delay2/1 -> HDL Counter/1
  Delay/1 -> Нахождение окрестности середины ЗИ/1(MagIn)
  Constant4/1 -> Relational Operator5/2
  Delay9/1 -> Switch/2
  Delay1/1 -> Delay6/1
  AngleIn/1 -> Delay1/1
  MagIn/1 -> Delay5/1
  Data Type Conversion1/1 -> Delay7/1, Gain1/1
  Gain1/1 -> Unit Delay Enabled2/1
  ValidIn/1 -> Delay2/1
  HDL Counter2/1 -> Relational Operator5/1
  Delay5/1 -> Задержка максимального значения/1(AmpIn), Delay/1
  Задержка максимального значения/1("MagMax ") -> Нахождение окрестности середины ЗИ/2(MagMax)
  Compare To Constant/1 -> Нахождение окрестности середины ЗИ/3("Reset "), Задержка максимального значения/2("Reset ")
  Нахождение окрестности середины ЗИ/1(MiddleRdEn) -> HDL Counter1/2, Logical Operator4/1, HDL Counter2/2, Switch1/2, Delay9/1, Unit Delay Enabled1/2, Logical Operator1/1
  HDL Counter1/1 -> Compare To Constant1/1
  Unit Delay Enabled/1 -> Scope1/1
  Delay4/1 -> Add2/2, Unit Delay Enabled1/1
  Add2/1 -> Delay10/1
  Delay10/1 -> Data Type Conversion2/1
  Gain2/1 -> Unit Delay Enabled/1
  Data Type Conversion2/1 -> Gain2/1, Add2/1
  Compare To Constant1/1 -> Unit Delay Enabled/2
  Logical Operator1/1 -> HDL Counter1/1

== system OFDMTxRx221121/LTE_Detector_HDL/Frequency_Estimation/Cyclic_Prefix_Correlator ==
  dataIn : Inport
  Delay1 : Delay  DelayLength=1  InitialCondition=0  UseCircularBuffer=on
  Delay2 : Delay  DelayLength=1024  InitialCondition=0
  Delay3 : Delay  DelayLength=1  InitialCondition=0  UseCircularBuffer=on
  Delay5 : Delay  DelayLength=1  InitialCondition=0  UseCircularBuffer=on
  Moving_Average : Subsystem
  Product : Product  OutDataTypeStr=fixdt(1,24,23)  RndMeth=Round
  Slot_Average : Subsystem
  complexConj : Math  Operator=conj  SaturateOnIntegerOverflow=on
  corrOut : Outport
  wires:
  Product/1 -> Delay5/1
  Delay3/1 -> Product/2
  Delay2/1 -> complexConj/1
  Slot_Average/1(dataOut) -> corrOut/1
  complexConj/1 -> Delay3/1
  Delay1/1 -> Product/1
  dataIn/1 -> Delay2/1, Delay1/1
  Delay5/1 -> Moving_Average/1(dataIn)
  Moving_Average/1(dataOut) -> Slot_Average/1(dataIn)

== system OFDMTxRx221121/LTE_Detector_HDL/Frequency_Estimation/Rect_to_Polar ==
  dataIn : Inport
  Complex to Magnitude-Angle HDL Optimized : dspmathops/Complex to Magnitude-Angle HDL Optimized  NumIterationsSource=Auto  NumIterations=16  OutputFormat=Magnitude and angle  AngleFormat=Normalized  ScaleOutput=on  SimulateUsing=Code generation
      settings: SourceProductName=DSP System Toolbox  SourceProductBaseCode=DS
  Constant : Constant  OutDataTypeStr=boolean  SampleTime=simParams.TsRx
  Delay1 : Delay  InitialCondition=0  UseCircularBuffer=on
  Delay2 : Delay  DelayLength=1  InitialCondition=0  UseCircularBuffer=on
  Delay3 : Delay  DelayLength=1  InitialCondition=0  UseCircularBuffer=on
  Delay4 : Delay  DelayLength=1  InitialCondition=0  UseCircularBuffer=on
  Delay5 : Delay  InitialCondition=0  UseCircularBuffer=on
  Gain : Gain  Gain=0.5  OutDataTypeStr=fixdt(1,27,27)
  Signal Specification1 : SignalSpecification  Dimensions=1
  magOut : Outport
  angleOut : Outport  Port=2
  validOut : Outport  Port=3
  wires:
  Gain/1 -> angleOut/1
  dataIn/1 -> Signal Specification1/1
  Constant/1 -> Delay1/1
  Delay5/1 -> Complex to Magnitude-Angle HDL Optimized/1
  Delay1/1 -> Complex to Magnitude-Angle HDL Optimized/2
  Delay2/1 -> magOut/1
  Delay3/1 -> Gain/1
  Delay4/1 -> validOut/1
  Complex to Magnitude-Angle HDL Optimized/1 -> Delay2/1
  Complex to Magnitude-Angle HDL Optimized/3 -> Delay4/1
  Complex to Magnitude-Angle HDL Optimized/2 -> Delay3/1
  Signal Specification1/1 -> Delay5/1

== system OFDMTxRx221121/LTE_Detector_HDL/Frequency_Estimation1/Angle_Filter ==
  note: This subsystem implements a 1-pole IIR filter to perform further averaging of the correlation angle results. The filter's gain is normalized to 0dB and an efficient implementation which requires only 1 multiplier is used.
  angleIn : Inport
  en : Inport  Port=2
  Add : Sum  Inputs=|-+
  Add1 : Sum  Inputs=|-+
  Data Type Conversion : DataTypeConversion
  Data Type Conversion1 : DataTypeConversion
  Delay1 : Delay  DelayLength=1  InitialCondition=0  UseCircularBuffer=on
  Delay2 : Delay  DelayLength=1  InitialCondition=0  UseCircularBuffer=on
  Delay3 : Delay  DelayLength=1  InitialCondition=0  UseCircularBuffer=on
  Gain : Gain  Gain=2^-2  OutDataTypeStr=Inherit: Same as input
  Unit Delay Enabled : simulink_need_slupdate/Unit Delay Enabled  vinit=0.0  tsamp=-1
      settings: SourceProductName=Simulink  SourceProductBaseCode=SL
  angleOut : Outport
  wires:
  angleIn/1 -> Delay2/1
  Add/1 -> Data Type Conversion/1
  Gain/1 -> Add1/1
  Unit Delay Enabled/1 -> Add1/2, Delay1/1, Add/2
  Add1/1 -> Data Type Conversion1/1
  en/1 -> Delay3/1
  Delay1/1 -> angleOut/1
  Delay2/1 -> Add/1
  Delay3/1 -> Unit Delay Enabled/2
  Data Type Conversion/1 -> Gain/1
  Data Type Conversion1/1 -> Unit Delay Enabled/1

== system OFDMTxRx221121/LTE_Detector_HDL/Frequency_Estimation1/Angle_at_Maximum ==
  magIn : Inport
  angleIn : Inport  Port=2
  validIn : Inport  Port=3
  Compare To Constant : simulink/Logic and Bit Operations/Compare To Constant  relop===  const=0  OutDataTypeStr=boolean
  Delay{1..3,5} (4 alike) : Delay  DelayLength=1  InitialCondition=0  UseCircularBuffer=on
  Delay4 : Delay  DelayLength=128  InitialCondition=0  UseCircularBuffer=on
  Delay6 : Delay  DelayLength=128  InitialCondition=0  UseCircularBuffer=on
  HDL Counter : hdlsllib/Sources/HDL Counter  CountType=Count limited  CountInit=0  CountStep=1  CountMax=1152  CountFromType=Initial value  CountFrom=0  CountResetPort=off  CountLoadPort=off  CountEnbPort=on  CountDirPort=off  CountDataType=Unsigned  CountWordLen=11  CountFracLen=0  CountSampTime=1
      settings: SourceProductBaseCode=HD
  Logical Operator : Logic  Operator=OR  IconShape=distinctive  AllPortsSameDT=off  OutDataTypeStr=boolean
  Relational Operator : RelationalOperator  Operator=>  OutDataTypeStr=boolean  RndMeth=Nearest
  Subsystem : Subsystem
  Unit Delay Enabled : simulink_need_slupdate/Unit Delay Enabled  vinit=0.0  tsamp=-1
      settings: SourceProductName=Simulink  SourceProductBaseCode=SL
  Unit Delay Enabled2 : simulink_need_slupdate/Unit Delay Enabled  vinit=0.0  tsamp=-1
      settings: SourceProductName=Simulink  SourceProductBaseCode=SL
  Средняя сумма 8 текущих отсчетов : Subsystem
  angleOut : Outport
  validOut : Outport  Port=2
  wires:
  Delay4/1 -> Subsystem/1(Amp)
  Unit Delay Enabled2/1 -> angleOut/1
  Compare To Constant/1 -> Logical Operator/2
  Logical Operator/1 -> Unit Delay Enabled/2
  Delay3/1 -> validOut/1
  Средняя сумма 8 текущих отсчетов/1(dataOut) -> Unit Delay Enabled2/1
  Unit Delay Enabled/1 -> Subsystem/2(MaxAmp), Relational Operator/2
  Delay2/1 -> HDL Counter/1
  Delay5/1 -> Relational Operator/1, Unit Delay Enabled/1, Delay4/1
  Delay1/1 -> Delay6/1
  validIn/1 -> Delay2/1
  Relational Operator/1 -> Logical Operator/1
  angleIn/1 -> Delay1/1
  HDL Counter/1 -> Compare To Constant/1
  magIn/1 -> Delay5/1
  Delay6/1 -> Средняя сумма 8 текущих отсчетов/1(dataIn)
  Subsystem/2(LastSampOfWindow) -> Delay3/1, Unit Delay Enabled2/2

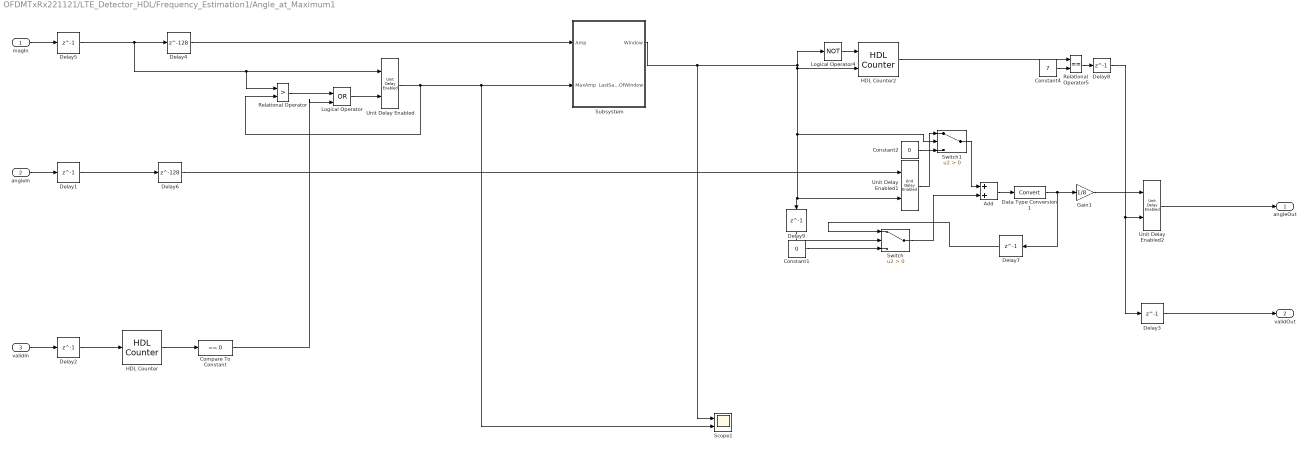
== system OFDMTxRx221121/LTE_Detector_HDL/Frequency_Estimation1/Angle_at_Maximum1 ==
  magIn : Inport
  angleIn : Inport  Port=2
  validIn : Inport  Port=3
  Add : Sum
  Compare To Constant : simulink/Logic and Bit Operations/Compare To Constant  relop===  const=0  OutDataTypeStr=boolean
  Constant1 : Constant  Value=0
  Constant2 : Constant  Value=0
  Constant4 : Constant  Value=7
  Data Type Conversion1 : DataTypeConversion
  Delay{1..3,5,7..9} (7 alike) : Delay  DelayLength=1  InitialCondition=0  UseCircularBuffer=on
  Delay4 : Delay  DelayLength=128  InitialCondition=0  UseCircularBuffer=on
  Delay6 : Delay  DelayLength=128  InitialCondition=0  UseCircularBuffer=on
  Gain1 : Gain  Gain=1/8
  HDL Counter : hdlsllib/Sources/HDL Counter  CountType=Count limited  CountInit=0  CountStep=1  CountMax=1152  CountFromType=Initial value  CountFrom=0  CountResetPort=off  CountLoadPort=off  CountEnbPort=on  CountDirPort=off  CountDataType=Unsigned  CountWordLen=11  CountFracLen=0  CountSampTime=1
      settings: SourceProductBaseCode=HD
  HDL Counter2 : hdlsllib/Sources/HDL Counter  CountType=Count limited  CountInit=0  CountStep=1  CountMax=7  CountFromType=Initial value  CountFrom=0  CountResetPort=on  CountLoadPort=off  CountEnbPort=on  CountDirPort=off  CountDataType=Unsigned  CountWordLen=3  CountFracLen=0  CountSampTime=1
      settings: SourceProductBaseCode=HD
  Logical Operator : Logic  Operator=OR  IconShape=distinctive  AllPortsSameDT=off  OutDataTypeStr=boolean
  Logical Operator4 : Logic  Operator=NOT  IconShape=distinctive  AllPortsSameDT=off  OutDataTypeStr=boolean
  Relational Operator : RelationalOperator  Operator=>  OutDataTypeStr=boolean  RndMeth=Nearest
  Relational Operator5 : RelationalOperator  Operator===  OutDataTypeStr=boolean  RndMeth=Nearest
  Scope1 : Scope  NumInputPorts=2
  Subsystem : Subsystem
  Switch : Switch  Criteria=u2 > Threshold
  Switch1 : Switch  Criteria=u2 > Threshold
  Unit Delay Enabled : simulink_need_slupdate/Unit Delay Enabled  vinit=0.0  tsamp=-1
      settings: SourceProductName=Simulink  SourceProductBaseCode=SL
  Unit Delay Enabled1 : simulink_need_slupdate/Unit Delay Enabled  vinit=0.0  tsamp=-1
      settings: SourceProductName=Simulink  SourceProductBaseCode=SL
  Unit Delay Enabled2 : simulink_need_slupdate/Unit Delay Enabled  vinit=0.0  tsamp=-1
      settings: SourceProductName=Simulink  SourceProductBaseCode=SL
  angleOut : Outport
  validOut : Outport  Port=2
  wires:
  Delay4/1 -> Subsystem/1(Amp)
  Unit Delay Enabled1/1 -> Switch1/1
  Unit Delay Enabled2/1 -> angleOut/1
  Compare To Constant/1 -> Logical Operator/2
  Logical Operator/1 -> Unit Delay Enabled/2
  Constant1/1 -> Switch/3
  Delay7/1 -> Switch/1
  Delay3/1 -> validOut/1
  Constant2/1 -> Switch1/3
  Gain1/1 -> Unit Delay Enabled2/1
  Subsystem/1(Window) -> Scope1/1, Switch1/2, Delay9/1, Unit Delay Enabled1/2, HDL Counter2/2, Logical Operator4/1
  Delay9/1 -> Switch/2
  Unit Delay Enabled/1 -> Scope1/2, Subsystem/2(MaxAmp), Relational Operator/2
  Data Type Conversion1/1 -> Delay7/1, Gain1/1
  Logical Operator4/1 -> HDL Counter2/1
  Switch1/1 -> Add/1
  Add/1 -> Data Type Conversion1/1
  Relational Operator5/1 -> Delay8/1
  Delay2/1 -> HDL Counter/1
  HDL Counter2/1 -> Relational Operator5/1
  Constant4/1 -> Relational Operator5/2
  Delay8/1 -> Unit Delay Enabled2/2, Delay3/1
  Delay6/1 -> Unit Delay Enabled1/1
  Delay5/1 -> Relational Operator/1, Unit Delay Enabled/1, Delay4/1
  Delay1/1 -> Delay6/1
  validIn/1 -> Delay2/1
  Relational Operator/1 -> Logical Operator/1
  angleIn/1 -> Delay1/1
  HDL Counter/1 -> Compare To Constant/1
  magIn/1 -> Delay5/1
  Switch/1 -> Add/2
